simulink model "test_5"  (R2017b)
settings: Solver=VariableStepAuto  StartTime=0.0  StopTime=3  RelTol=1e-3
undefined symbols (not defined in the file): Cwy1, Cwy2, Jyy, k1_k, k2_k, K_thruster, kc, lambda55, T_thruster
settings Model: Creator=Eugene  LastModifiedBy=Eugene

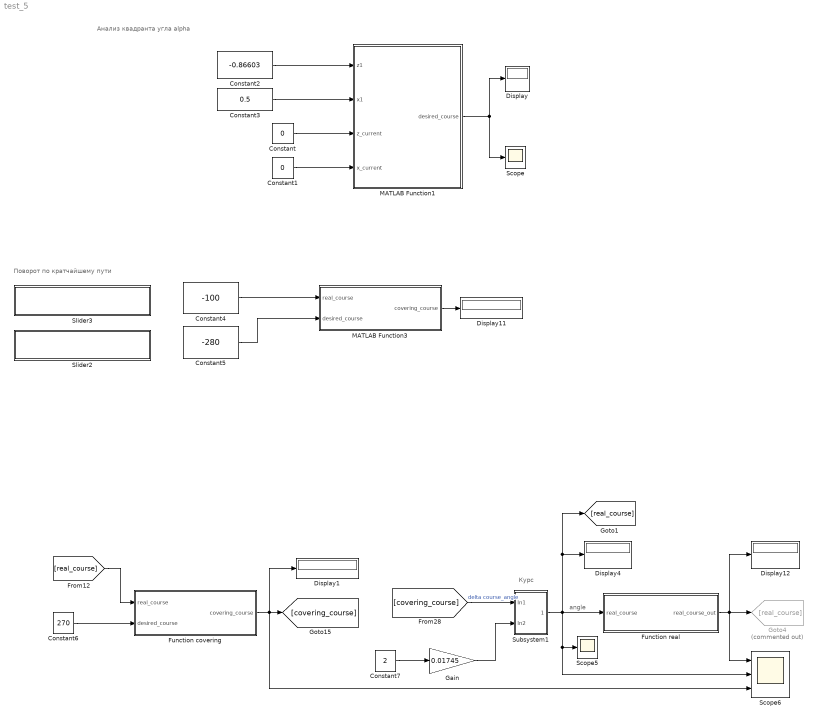
== system test_5 ==
  note: Поворот по кратчайшему пути
  note: Анализ квадранта угла alpha
  note: Курс
  note: angle
  Constant : Constant  Value=0
  Constant1 : Constant  Value=0
  Constant2 : Constant  Value=-0.86603
  Constant3 : Constant  Value=0.5
  Constant4 : Constant  Value=-100
  Constant5 : Constant  Value=-280
  Constant6 : Constant  Value=270
  Constant7 : Constant  Value=2
  Display{,1,4,11..12} (5 alike) : Display
  Function covering : MATLAB Function  TreatAsAtomicUnit=on
  Function real : MATLAB Function  TreatAsAtomicUnit=on
  Gain : Gain  Gain=0.01745
  Goto4 : Goto  Commented=on  GotoTag=real_course
  MATLAB Function1 : MATLAB Function  TreatAsAtomicUnit=on
  MATLAB Function3 : MATLAB Function  TreatAsAtomicUnit=on
  Scope : Scope
  Scope5 : Scope
  Scope6 : Scope  NumInputPorts=3
  Slider2 : Subsystem  DialogController=hmiCreateDDGDialog  IsWebBlock=on  mask(MWDashboardBlock){webBlockId=beae14a9-6052-4aa7-916a-4f04d7c05d55, webBlockType=slider, ShowInLibBrowser=on, ShowInitialText=on, HMISrcModelName=test_5}
      mask prompts: webBlockId "WebBlock Id"; webBlockType "WebBlock Type"; HMISrcModelName "Source Model"
      mask help: SimulinkHMI:dialogs:SliderDialogDesc
      mask Help: helpview([docroot '/mapfiles/simulink.map'], 'hmi_slider')
      mask Display:
      | if strcmp(get_param(bdroot(gcb),'BlockDiagramType'), 'library')
      |     image([(matlabroot) '/toolbox/simulink/hmi/icons/Slider.png']);
      | end
  Slider3 : Subsystem  DialogController=hmiCreateDDGDialog  IsWebBlock=on  mask(MWDashboardBlock){webBlockId=003fc597-b61a-4663-9dbd-5e54f20fd45b, webBlockType=slider, ShowInLibBrowser=on, ShowInitialText=on, HMISrcModelName=test_5}
      mask prompts: webBlockId "WebBlock Id"; webBlockType "WebBlock Type"; HMISrcModelName "Source Model"
      mask help: SimulinkHMI:dialogs:SliderDialogDesc
      mask Help: helpview([docroot '/mapfiles/simulink.map'], 'hmi_slider')
      mask Display:
      | if strcmp(get_param(bdroot(gcb),'BlockDiagramType'), 'library')
      |     image([(matlabroot) '/toolbox/simulink/hmi/icons/Slider.png']);
      | end
  Subsystem1 : Subsystem
  wires:
  MATLAB Function1/1(desired_course) -> Scope/1, Display/1
  Constant1/1 -> MATLAB Function1/4(x_current)
  Constant/1 -> MATLAB Function1/3(z_current)
  Constant3/1 -> MATLAB Function1/2(x1)
  MATLAB Function3/1(covering_course) -> Display11/1
  Constant4/1 -> MATLAB Function3/1(real_course)
  Constant5/1 -> MATLAB Function3/2(desired_course)
  [real_course] -> Function covering/1(real_course)
  Function covering/1(covering_course) -> Scope6/3, Display1/1, [covering_course]
  Subsystem1/1(Out1) -> Scope6/2, Scope5/1, [real_course], Display4/1, Function real/1(real_course)
  [covering_course] -> Subsystem1/1(In1)  "delta course_angle"
  Function real/1(real_course_out) -> Scope6/1, Goto4/1, Display12/1
  Constant7/1 -> Gain/1
  Gain/1 -> Subsystem1/2(In2)
  Constant6/1 -> Function covering/2(desired_course)
  Constant2/1 -> MATLAB Function1/1(z1)

== system test_5/Slider2 ==

== system test_5/Slider3 ==

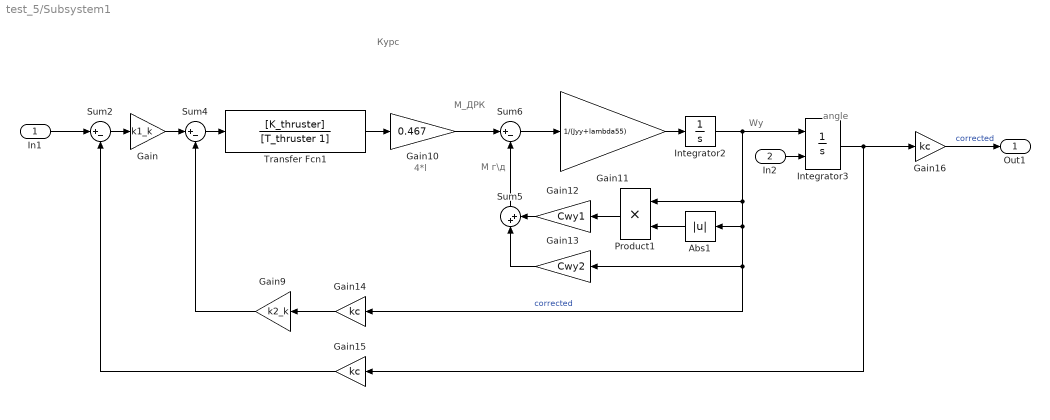
== system test_5/Subsystem1 ==
  note: Курс
  note: Wy
  note: M_ДРК
  note: 4*l
  note: angle
  note: M г\д
  In1 : Inport
  In2 : Inport  Port=2
  Abs1 : Abs
  Gain : Gain  Gain=k1_k
  Gain10 : Gain  Gain=0.467
  Gain11 : Gain  Gain=1/(Jyy+lambda55)
  Gain12 : Gain  Gain=Cwy1
  Gain13 : Gain  Gain=Cwy2
  Gain14 : Gain  Gain=kc
  Gain15 : Gain  Gain=kc
  Gain16 : Gain  Gain=kc
  Gain9 : Gain  Gain=k2_k
  Integrator2 : Integrator
  Integrator3 : Integrator  InitialConditionSource=external  InitialCondition=1.5708
  Product1 : Product
  Sum2 : Sum  Inputs=|+-
  Sum4 : Sum  Inputs=|+-
  Sum5 : Sum  Inputs=|++
  Sum6 : Sum  Inputs=|+-
  Transfer Fcn1 : TransferFcn  Numerator=[K_thruster]  Denominator=[T_thruster 1]
  Out1 : Outport
  wires:
  Gain12/1 -> Sum5/2
  Gain10/1 -> Sum6/1
  Product1/1 -> Gain12/1
  Gain11/1 -> Integrator2/1
  Gain9/1 -> Sum4/2
  Gain/1 -> Sum4/1
  Transfer Fcn1/1 -> Gain10/1
  Sum6/1 -> Gain11/1
  Gain14/1 -> Gain9/1
  Gain15/1 -> Sum2/2
  Gain13/1 -> Sum5/1
  Abs1/1 -> Product1/2
  Sum5/1 -> Sum6/2
  Integrator2/1 -> Gain14/1, Gain13/1, Abs1/1, Product1/1, Integrator3/1  "corrected"
  Sum2/1 -> Gain/1
  Integrator3/1 -> Gain16/1, Gain15/1
  Sum4/1 -> Transfer Fcn1/1
  In1/1 -> Sum2/1
  Gain16/1 -> Out1/1  "corrected"
  In2/1 -> Integrator3/2

== matlab function test_5/Function covering ==
  data: real_course input; desired_course input; covering_course output
function covering_course   = fcn(real_course, desired_course)

    % предстоит повернуться более чем на 180 градусов
    %if abs(desired_course - real_course) > 180
    %    covering_course = desired_course - 360 - real_course;
    %elseif desired_course < real_course
    %    covering_course = desired_course - real_course;
    %else    
    %    covering_course = desired_course;
    %end
    
    if abs(desired_course - real_course) > 180
        
        if desired_course > 180
            covering_course = desired_course - 360;
        elseif desired_course < -180
            covering_course = 360 + desired_course;
        else
            covering_course = desired_course;
        end
    else
        covering_course = desired_course;
    end
end

== matlab function test_5/MATLAB Function1 ==
  data: z1 input; x1 input; z_current input; desired_course output; x_current input
function desired_course = fcn(z1, x1, z_current, x_current)

delta_x = x1 - x_current;
delta_z = z1 - z_current;

%1
if (delta_x >= 0) && (delta_z >= 0)
    desired_course = 57.2958*atan(delta_z / delta_x);
%2    
elseif (delta_x >= 0) && (delta_z < 0)
    desired_course = 360 - 57.2958*atan( abs(delta_z) / delta_x);
%3    
elseif (delta_x < 0) && (delta_z < 0)    
    desired_course = 180 + 57.2958*atan(abs(delta_z) / abs(delta_x));
    
elseif (delta_x < 0) && (delta_z >= 0)    
    desired_course = 180 - 57.2958*atan( delta_z / abs(delta_x));   
    
else 
    desired_course = -1;
   
end

== matlab function test_5/MATLAB Function3 ==
  data: real_course input; desired_course input; covering_course output
function covering_course   = fcn(real_course, desired_course)

    % Поворот по кратчайшему пути
    if abs(desired_course - real_course) > 180
        covering_course = desired_course - 360 - real_course;
    else
        covering_course = desired_course;
    end

end

== matlab function test_5/Function real ==
  data: real_course input; real_course_out output
function real_course_out   = fcn(real_course)

    % Приводим к стандарту
    if real_course < 0
        real_course_out = 360 - abs(real_course);
    elseif real_course >= 360
        real_course_out = real_course - 360;
    else    
        real_course_out = real_course;
    end

end
